simulink model "HybridIntegrationEemshaven"  (R2022b)
settings: Solver=VariableStepAuto  StartTime=0.0  StopTime=1757.5  RelTol=1e-3
undefined symbols (not defined in the file): reactiveCompensationCapacitance
libraries: ee_lib x8, nesl_utility x4, fl_lib x2, spspowerguiLib x1
settings Model: Creator=anton  LastModifiedBy=andreas
settings SolverCC: AlgebraicLoopSolver=TrustRegion
settings DebuggingCC: UnconnectedInputMsg=warning  UnconnectedOutputMsg=warning  UnconnectedLineMsg=warning  SFMachineParentedDataDiag=warning
settings ModelReferenceCC: EnableRefExpFcnMdlSchedulingChecks=on
settings RTWCC: DLArmComputeVersion=19.05

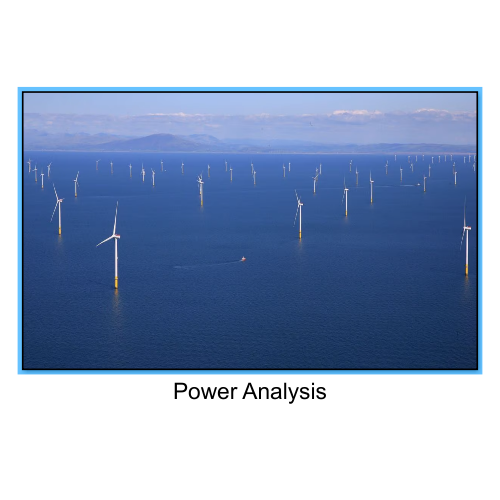
[thumbnail: Simulink's stored preview of the top-level diagram]
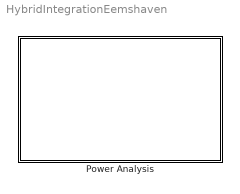
== system HybridIntegrationEemshaven ==
  Power Analysis : Subsystem
      mask Display: image('PowerAnalysis.PNG'); % Use "Edit Image" on toolstrip to change.

== system HybridIntegrationEemshaven/Power Analysis ==
  Ocean Battery : Subsystem
      mask Display: image('OceanBattery.jpg'); % Use "Edit Image" on toolstrip to change.
  Panels Input Data : Subsystem
      mask Display: image('PanelsInputData.jpg'); % Use "Edit Image" on toolstrip to change.
  Production Modules : Subsystem
      mask Display: image('ProductionModules.png'); % Use "Edit Image" on toolstrip to change.
  Scope5 : Scope
  Wave Power Input Data : Subsystem
      mask Display: image('Waves.jpg'); % Use "Edit Image" on toolstrip to change.
  powergui : spspowerguiLib/powergui  Priority=1  SimulationMode=Discrete phasor  SampleTime=0.05  frequency=60  Iterations=50  frequencyindice=60  Pbase=100e6  ErrMax=1e-4  UnitsV=kV  UnitsW=MW  buscounter=0  FunctionMessages=off  echomessages=off  EnableUseOfTLC=off  CurrentSourceSwitches=off  DisableSnubberDevices=off  DisableRonSwitches=off  DisableVfSwitches=off  DisplayEquations=off  AutomaticDiscreteSolvers=off  SolverType=Tustin/Backward Euler (TBE)  Interpol=off  ExternalGateDelay=off  methode=off  Ts=100  x0status=blocks  SPID=on  SwTol=0  HookPort=off  NonlinearTolerance=1e-4  nMaxIteration=100  ContinueOnMaxIteration=off  RestoreLinks=warning  ResistiveCurrentMeasurement=off  Frange=[0:2:500]  Ylog=off  Xlog=on  ShowGrid=off  save=off  variable=ZData  structure=0  ZoomFFT=off  StartTime=0.0  cycles=1  DisplayStyle=1  fundamental=60  FreqAxis=off  MaxFrequency=1000  frequencyindicesteady=1  RmsSteady=1  display=off
  wires:
  Production Modules/1("Total Power (Wind, Sun, Wave)") -> Ocean Battery/1(Input), Scope5/1

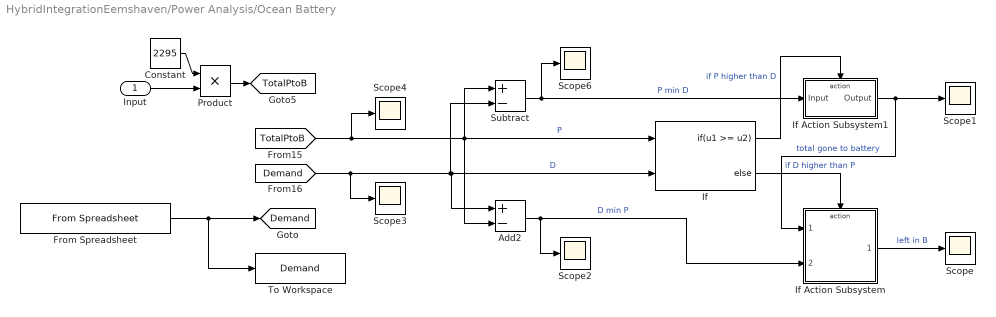
== system HybridIntegrationEemshaven/Power Analysis/Ocean Battery ==
  Input : Inport
  Add2 : Sum  Inputs=+-
  Constant : Constant  Value=2295
  From Spreadsheet : FromSpreadsheet  FileName=Copy of DemandSheet5.xlsx  SheetName=Sheet5  Range=A2:B35654  SampleTime=0.05
  If : If  NumInputs=2  IfExpression=u1 >= u2
  If Action Subsystem : Subsystem  TreatAsAtomicUnit=on
  If Action Subsystem1 : Subsystem  TreatAsAtomicUnit=on
  Product : Product
  Scope{,1..4,6} (6 alike) : Scope
  Subtract : Sum  Inputs=+-
  To Workspace : ToWorkspace  VariableName=Demand  SampleTime=-1
      settings: Save2DSignal=2-D array (concatenate along first dimension)
  tag scope: Demand=global, TotalPtoB=global
  wires:
  [TotalPtoB] -> Scope4/1, Subtract/1, If/1, Add2/2  "P"
  If Action Subsystem/1(Output) -> Scope/1  "left in B"
  Constant/1 -> Product/1
  [Demand] -> Add2/1, If/2, Subtract/2, Scope3/1  "D"
  Add2/1 -> If Action Subsystem/2(D min P), Scope2/1  "D min P"
  Subtract/1 -> If Action Subsystem1/1(Input), Scope6/1  "P min D"
  If Action Subsystem1/1(Output) -> If Action Subsystem/1(Total to battery), Scope1/1  "total gone to battery"
  From Spreadsheet/1 -> To Workspace/1, [Demand]
  If/2 -> If Action Subsystem/Action  "if D higher than P"
  Product/1 -> [TotalPtoB]
  Input/1 -> Product/2
  If/1 -> If Action Subsystem1/Action  "if P higher than D"

== system HybridIntegrationEemshaven/Power Analysis/Panels Input Data ==
  From Spreadsheet : FromSpreadsheet  FileName=EemshavenVoltageSheet4.xlsx  SheetName=Sheet4  Range=A2:B35300  SampleTime=0.05
  From Spreadsheet1 : FromSpreadsheet  FileName=EemshavenSunIrradSheet5.xlsx  SheetName=Sheet5  Range=A2:B35300  SampleTime=0.05
  Scope1 : Scope
  Scope2 : Scope
  tag scope: G=global, Voltage=global
  wires:
  From Spreadsheet1/1 -> Scope1/1, [G]
  From Spreadsheet/1 -> [Voltage], Scope2/1

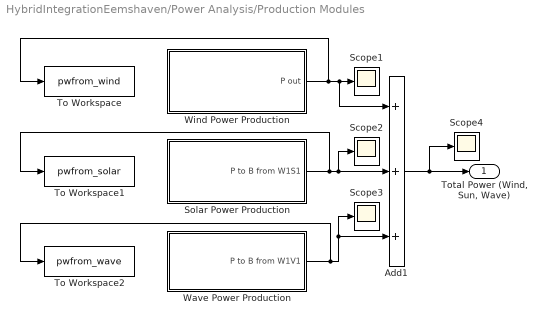
== system HybridIntegrationEemshaven/Power Analysis/Production Modules ==
  Add1 : Sum  Inputs=+++
  Scope{1..4} (4 alike) : Scope
  Solar Power Production : Subsystem
      mask Display: image('Panels.jpg'); % Use "Edit Image" on toolstrip to change.
  To Workspace : ToWorkspace  VariableName=pwfrom_wind  SampleTime=0.05
      settings: Save2DSignal=2-D array (concatenate along first dimension)
  To Workspace1 : ToWorkspace  VariableName=pwfrom_solar  SampleTime=-1
      settings: Save2DSignal=2-D array (concatenate along first dimension)
  To Workspace2 : ToWorkspace  VariableName=pwfrom_wave  SampleTime=-1
      settings: Save2DSignal=2-D array (concatenate along first dimension)
  Wave Power Production : Subsystem
      mask Display: image('WavePower.jpeg'); % Use "Edit Image" on toolstrip to change.
  Wind Power Production : Subsystem
      mask Display: image('WindPower.PNG'); % Use "Edit Image" on toolstrip to change.
  "Total Power (Wind, Sun, Wave)" : Outport
  wires:
  Add1/1 -> "Total Power (Wind, Sun, Wave)"/1, Scope4/1
  Solar Power Production/1(P to B from W1S1) -> To Workspace1/1, Add1/2, Scope2/1
  Wind Power Production/1(P out) -> Add1/1, Scope1/1, To Workspace/1
  Wave Power Production/1(P to B from W1V1) -> To Workspace2/1, Scope3/1, Add1/3

== system HybridIntegrationEemshaven/Power Analysis/Wave Power Input Data ==
  From Spreadsheet : FromSpreadsheet  FileName=EemshavenWavePerBuoySheet5.xlsx  SheetName=Sheet5  Range=A2:B35533  SampleTime=0.05
  tag scope: WavePower=global
  wires:
  From Spreadsheet/1 -> [WavePower]

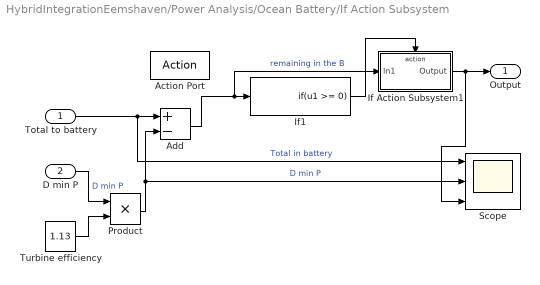
== system HybridIntegrationEemshaven/Power Analysis/Ocean Battery/If Action Subsystem ==
  Total to battery : Inport
  D min P : Inport  Port=2
  Action Port : ActionPort  ActionPortLabel=else
  Add : Sum  Inputs=+-
  If Action Subsystem1 : Subsystem  TreatAsAtomicUnit=on
  If1 : If  IfExpression=u1 >= 0  ShowElse=off
  Product : Product
  Scope : Scope  NumInputPorts=3
  Turbine efficiency : Constant  Value=1.13
  Output : Outport
  wires:
  D min P/1 -> Product/1  "D min P"
  Product/1 -> Add/2, Scope/2  "D min P"
  Total to battery/1 -> Add/1, Scope/1  "Total in battery"
  Turbine efficiency/1 -> Product/2
  If1/1 -> If Action Subsystem1/Action
  Add/1 -> If Action Subsystem1/1(In1), If1/1  "remaining in the B"
  If Action Subsystem1/1(Output) -> Scope/3, Output/1

== system HybridIntegrationEemshaven/Power Analysis/Ocean Battery/If Action Subsystem1 ==
  Input : Inport
  Action Port : ActionPort  ActionPortLabel=if(u1 >= u2)
  If Action Subsystem1 : Subsystem  TreatAsAtomicUnit=on
  If1 : If  IfExpression=u1 <= 2.44e+6  ShowElse=off
  Scope : Scope
  Output : Outport
  wires:
  Input/1 -> If Action Subsystem1/1(Input), If1/1  "To Battery"
  If Action Subsystem1/1(Output) -> Scope/1, Output/1
  If1/1 -> If Action Subsystem1/Action

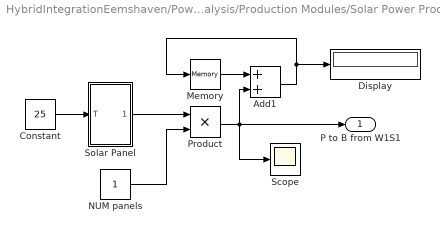
== system HybridIntegrationEemshaven/Power Analysis/Production Modules/Solar Power Production ==
  Add1 : Sum
  Constant : Constant  Value=25
  Display : Display
  Memory : Memory
  NUM panels : Constant
  Product : Product
  Scope : Scope
  Solar Panel : Subsystem
  P to B from W1S1 : Outport
  wires:
  Constant/1 -> Solar Panel/1(T)
  Product/1 -> Scope/1, Add1/2, P to B from W1S1/1
  NUM panels/1 -> Product/2
  Solar Panel/1(Out1) -> Product/1
  Add1/1 -> Memory/1, Display/1
  Memory/1 -> Add1/1

== system HybridIntegrationEemshaven/Power Analysis/Production Modules/Wave Power Production ==
  NUM_buoys : Constant
  Product : Product
  Scope16 : Scope
  P to B from W1V1 : Outport
  wires:
  NUM_buoys/1 -> Product/1
  [WavePower] -> Product/2
  Product/1 -> Scope16/1, P to B from W1V1/1

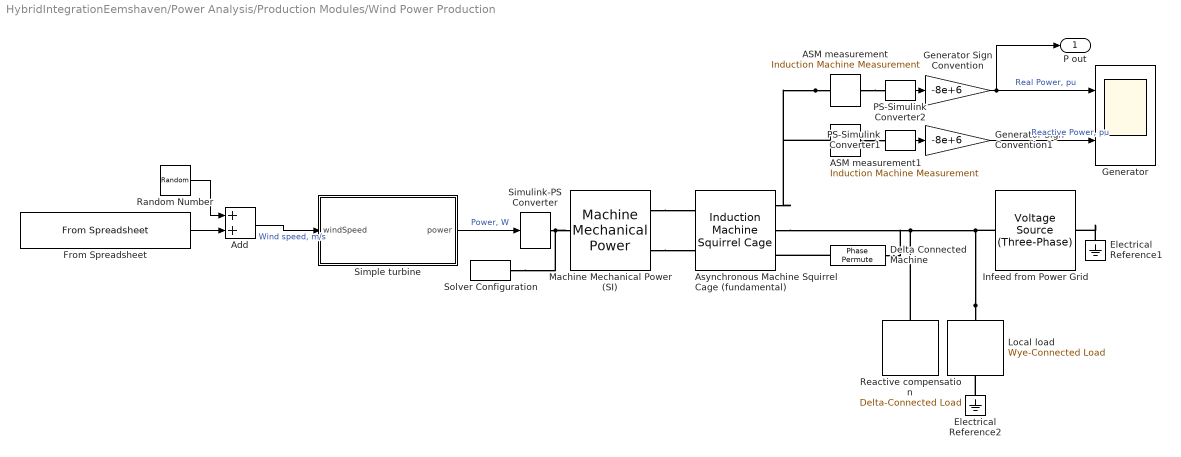
== system HybridIntegrationEemshaven/Power Analysis/Production Modules/Wind Power Production ==
  ASM measurement : ee_lib/Electromechanical/Asynchronous/Induction Machine Measurement  output_idx=11
      settings: InternalSimscapePortConfiguration="{\"Bottom\":[],\"Left\":[{\"id\":\"pu_input\",\"label\":\"pu\",\"type\":\"input\"}],\"Right\":[{\"id\":\"pu_output\",\"label\":\"o\",\"type\":\"output\"}],\"Top\":[]}"
  ASM measurement1 : ee_lib/Electromechanical/Asynchronous/Induction Machine Measurement  output_idx=12
      settings: InternalSimscapePortConfiguration="{\"Bottom\":[],\"Left\":[{\"id\":\"pu_input\",\"label\":\"pu\",\"type\":\"input\"}],\"Right\":[{\"id\":\"pu_output\",\"label\":\"o\",\"type\":\"output\"}],\"Top\":[]}"
  Add : Sum
  Asynchronous Machine Squirrel Cage (fundamental) : ee_lib/Electromechanical/Asynchronous/Induction Machine Squirrel Cage  port_option=ee.enum.threePhasePort.composite  SRated=SRated V*A  VRated=VRated V  FRated=FRated Hz  nPolePairs=2  param_unit=ee.enum.unit.si  squirrel_cage=ee.enum.squirrelcage.Single  zero_sequence=ee.enum.park.zerosequence.include  initialization_option=ee.enum.asm.initialization.fluxvariables  Rs=0.25 Ohm  Xls=0.4 Ohm  pu_Rs=0.0258  pu_Lls=0.0413  Rrd=0.14 Ohm  Xlrd=0.41 Ohm  pu_Rrd=0.0145  pu_Llrd=0.0424  Rrd1=0.28 Ohm  Xlrd1=0.82 Ohm  Rrd2=0.28 Ohm  Xlrd2=0.82 Ohm  pu_Rrd1=0.0290  pu_Llrd1=0.0848  pu_Rrd2=0.0290  pu_Llrd2=0.0848  Xm=17 Ohm  pu_Lm=1.7562  X0=0.4 Ohm  pu_L0=0.0413  saturation_option=ee.enum.saturation.exclude  saturation_i=[0, 4, 9, 18, 25, 34, 50, 68, 95, 120] A  saturation_v=[0, 88, 154, 198, 220, 242, 264, 286, 308, 327] V  pu_saturation_i=[0, .176, .396, .792, 1.1, 1.496, 2.2, 2.992, 4.18, 5.28]  pu_saturation_v=[0, .4, .7, .9, 1, 1.1, 1.2, 1.3, 1.4, 1.4864]  connection_option=ee.enum.Connection.delta1  angular_position_specify=off  angular_position_priority=None  angular_position=0 deg  angular_position_nominal_specify=off  angular_position_nominal_unit=deg  angular_position_nominal_value=1  pu_psids_specify=off  pu_psids_priority=None  pu_psids=0  pu_psids_nominal_specify=off  pu_psids_nominal_unit=1  pu_psids_nominal_value=1  pu_psiqs_specify=off  pu_psiqs_priority=None  pu_psiqs=0  pu_psiqs_nominal_specify=off  pu_psiqs_nominal_unit=1  pu_psiqs_nominal_value=1  pu_psi0s_specify=off  pu_psi0s_priority=None  pu_psi0s=0  pu_psi0s_nominal_specify=off  pu_psi0s_nominal_unit=1  pu_psi0s_nominal_value=1  pu_psidr_specify=off  pu_psidr_priority=None  pu_psidr=0  pu_psidr_nominal_specify=off  pu_psidr_nominal_unit=1  pu_psidr_nominal_value=1  pu_psiqr_specify=off  pu_psiqr_priority=None  pu_psiqr=0  pu_psiqr_nominal_specify=off  pu_psiqr_nominal_unit=1  pu_psiqr_nominal_value=1  pu_psidr1_specify=off  pu_psidr1_priority=None  pu_psidr1=0  pu_psidr1_nominal_specify=off  pu_psidr1_nominal_unit=1  pu_psidr1_nominal_value=1  pu_psiqr1_specify=off  pu_psiqr1_priority=None  pu_psiqr1=0  pu_psiqr1_nominal_specify=off  pu_psiqr1_nominal_unit=1  pu_psiqr1_nominal_value=1  pu_psidr2_specify=off  pu_psidr2_priority=None  pu_psidr2=0  pu_psidr2_nominal_specify=off  pu_psidr2_nominal_unit=1  pu_psidr2_nominal_value=1  pu_psiqr2_specify=off  pu_psiqr2_priority=None  pu_psiqr2=0  pu_psiqr2_nominal_specify=off  pu_psiqr2_nominal_unit=1  pu_psiqr2_nominal_value=1  psids_specify=off  psids_priority=None  psids=0 Wb  psids_nominal_specify=off  psids_nominal_unit=Wb  psids_nominal_value=1  psiqs_specify=off  psiqs_priority=None  psiqs=0 Wb  psiqs_nominal_specify=off  psiqs_nominal_unit=Wb  psiqs_nominal_value=1  psi0s_specify=off  psi0s_priority=None  psi0s=0 Wb  psi0s_nominal_specify=off  psi0s_nominal_unit=Wb  psi0s_nominal_value=1  psidr_specify=off  psidr_priority=None  psidr=0 Wb  psidr_nominal_specify=off  psidr_nominal_unit=Wb  psidr_nominal_value=1  psiqr_specify=off  psiqr_priority=None  psiqr=0 Wb  psiqr_nominal_specify=off  psiqr_nominal_unit=Wb  psiqr_nominal_value=1  psidr1_specify=off  psidr1_priority=None  psidr1=0 Wb  psidr1_nominal_specify=off  psidr1_nominal_unit=Wb  psidr1_nominal_value=1  psiqr1_specify=off  psiqr1_priority=None  psiqr1=0 Wb  psiqr1_nominal_specify=off  psiqr1_nominal_unit=Wb  psiqr1_nominal_value=1  psidr2_specify=off  psidr2_priority=None  psidr2=0 Wb  psidr2_nominal_specify=off  psidr2_nominal_unit=Wb  psidr2_nominal_value=1  psiqr2_specify=off  psiqr2_priority=None  psiqr2=0 Wb  psiqr2_nominal_specify=off  psiqr2_nominal_unit=Wb  psiqr2_nominal_value=1  slip_specify=off  slip_priority=None  slip=0  slip_nominal_specify=off  slip_nominal_unit=1  slip_nominal_value=1  real_power_generated_specify=off  real_power_generated_priority=None  real_power_generated=0 W  real_power_generated_nominal_specify=off  real_power_generated_nominal_unit=W  real_power_generated_nominal_value=1  mechanical_power_consumed_specify=off  mechanical_power_consumed_priority=None  mechanical_power_consumed=0 W  mechanical_power_consumed_nominal_specify=off  mechanical_power_consumed_nominal_unit=W  mechanical_power_consumed_nominal_value=1  Tmeas=298.15 K  alpha=3.93e-3 1/K  alpha_cage=4.4e-3 1/K  stator_thermal_mass=100 J/K  rotor_thermal_mass=200 J/K  temperatureA_specify=off  temperatureA_priority=High  temperatureA=25 degC  temperatureA_nominal_specify=off  temperatureA_nominal_unit=degC  temperatureA_nominal_value=1  temperatureB_specify=off  temperatureB_priority=High  temperatureB=25 degC  temperatureB_nominal_specify=off  temperatureB_nominal_unit=degC  temperatureB_nominal_value=1  temperatureC_specify=off  temperatureC_priority=High  temperatureC=25 degC  temperatureC_nominal_specify=off  temperatureC_nominal_unit=degC  temperatureC_nominal_value=1  temperatureR_specify=off  temperatureR_priority=High  temperatureR=25 degC  temperatureR_nominal_specify=off  temperatureR_nominal_unit=degC  temperatureR_nominal_value=1
      settings: InternalSimscapePortConfiguration="{\"Bottom\":[],\"Left\":[{\"id\":\"R\",\"label\":\"R\",\"type\":\"foundation.mechanical.rotational.rotational\"},{\"id\":\"C\",\"label\":\"C\",\"type\":\"foundation.mechanical.rotational.rotational\"}],\"Right\":[{\"id\":\"pu_output\",\"label\":\"pu\",\"type\":\"output\"},{\"id\":\"N1\",\"label\":\"~1\",\"type\":\"foundation.electrical.three_phase\"},{\"id\":\"N2\",\"label\":\"~2\",\"type\":\"foundation.electrical.three_phase\"}],\"Top\":[]}"
  Delta Connected Machine : ee_lib/Connectors & References/Phase Permute
      settings: InternalSimscapePortConfiguration="{\"Bottom\":[],\"Left\":[{\"id\":\"N123\",\"label\":\"~123\",\"type\":\"foundation.electrical.three_phase\"}],\"Right\":[{\"id\":\"N231\",\"label\":\"~231\",\"type\":\"foundation.electrical.three_phase\"}],\"Top\":[]}"
  Electrical Reference1 : fl_lib/Electrical/Electrical Elements/Electrical Reference
  Electrical Reference2 : fl_lib/Electrical/Electrical Elements/Electrical Reference
  From Spreadsheet : FromSpreadsheet  FileName=EemshavenWindspeedSheet6.xlsx  SheetName=Sheet6  Range=A2:B35170  SampleTime=0.05
  Generator : Scope  NumInputPorts=2
  Generator Sign Convention : Gain  Gain=-8e+6
  Generator Sign Convention1 : Gain  Gain=-8e+6
  Infeed from Power Grid : ee_lib/Sources/Voltage Source (Three-Phase)  vline_rms=VRated V  shift=0 deg  freq=FRated Hz  impedance_option=0  SShortCircuit=1e6 V*A  XR=15  R=0.01 Ohm  L=3.97e-4 H  harmonic_option=0  harmonic_orders=[5, 7, 11, 13]  harmonic_ratios=[0.1, 0.1, 0.1, 0.1]  G_parasitic=0 1/Ohm  I_specify=off  I_priority=None  I=[ 0 0 0 ] A  I_nominal_specify=off  I_nominal_unit=A  I_nominal_value=1
  Local load : ee_lib/Passive/RLC Assemblies/Wye-Connected Load  parameterization=2  component_structure=1  component_structure_PQ=1  R=1 Ohm  L=0.001 H  C=1e-6 F  VRated=VRated V  FRated=60 Hz  P=75e3 W  Qpos=100 V*A  Qneg=-100 V*A  R_parasitic=1e-6 Ohm  G_parasitic=1e-6 1/Ohm  R_parasitic_PQ=1e-6 Ohm  G_parasitic_PQ=1e-6 1/Ohm  Vmag0=2.4e+4 V  Vang0=0 deg  Freq0=60 Hz  IL_specify=on  IL_priority=High  IL=[ 0 0 0 ] A  IL_nominal_specify=off  IL_nominal_unit=A  IL_nominal_value=1  VC_specify=on  VC_priority=High  VC=[ 0 0 0 ] V  VC_nominal_specify=off  VC_nominal_unit=V  VC_nominal_value=1
  Machine Mechanical Power (SI) : ee_lib/Electromechanical/Mechanical/Machine Mechanical Power  power_sign=-1  SRated=SRated V*A  FRated=FRated Hz  nPolePairs=2  inputUnit=ee.enum.unit.si  torque_factor=2  inertia_option=2  J=27548 kg*m^2  H=4 s*W/V/A  damper_option=2  D=39.0509 N*m/(rad/s)  pu_D=0.01  initialization_option=2  fMechanical0=30 Hz  fElectrical0=FRated Hz
      settings: InternalSimscapePortConfiguration="{\"Bottom\":[],\"Left\":[{\"id\":\"Pm\",\"label\":\"Pm\",\"type\":\"input\"}],\"Right\":[{\"id\":\"R\",\"label\":\"R\",\"type\":\"foundation.mechanical.rotational.rotational\"},{\"id\":\"C\",\"label\":\"C\",\"type\":\"foundation.mechanical.rotational.rotational\"}],\"Top\":[]}"
  PS-Simulink Converter1 : nesl_utility/PS-Simulink Converter  PhysicalDomain=network_engine_domain  SubClassName=ps_output  LeftPortType=input  RightPortType=output  PseudoPeriodic=off  Frequencies=[]  VectorFormat=1-D array  Unit=1  AffineConversion=off
  PS-Simulink Converter2 : nesl_utility/PS-Simulink Converter  PhysicalDomain=network_engine_domain  SubClassName=ps_output  LeftPortType=input  RightPortType=output  PseudoPeriodic=off  Frequencies=[]  VectorFormat=1-D array  Unit=1  AffineConversion=off
  Random Number : RandomNumber  Mean=5  Variance=3  SampleTime=0.05
  Reactive compensation : ee_lib/Passive/RLC Assemblies/Delta-Connected Load  parameterization=1  component_structure=3  component_structure_PQ=1  R=1 Ohm  L=0.001 H  C=reactiveCompensationCapacitance F  VRated=2.4e+4 V  FRated=60 Hz  P=1000 W  Qpos=100 V*A  Qneg=-100 V*A  R_parasitic=1e-6 Ohm  G_parasitic=1e-6 1/Ohm  R_parasitic_PQ=1e-6 Ohm  G_parasitic_PQ=1e-6 1/Ohm  Vmag0=2.4e+4 V  Vang0=0 deg  Freq0=60 Hz  IL_specify=on  IL_priority=High  IL=[ 0 0 0 ] A  IL_nominal_specify=off  IL_nominal_unit=A  IL_nominal_value=1  VC_specify=on  VC_priority=High  VC=[ 0 0 0 ] V  VC_nominal_specify=off  VC_nominal_unit=V  VC_nominal_value=1
      settings: InternalSimscapePortConfiguration="{\"Bottom\":[],\"Left\":[{\"id\":\"N\",\"label\":\"~\",\"type\":\"foundation.electrical.three_phase\"}],\"Right\":[],\"Top\":[]}"
  Simple turbine : MATLAB Function  TreatAsAtomicUnit=on  mask(Simple Turbine){ratedOutputPower=150e3, cutInSpeed=3, ratedOutputSpeed=12, cutOutSpeed=23}
      mask prompts: ratedOutputPower "Rated output power, W"; cutInSpeed "Cut-in speed, m/s"; ratedOutputSpeed "Rated output speed, m/s"; cutOutSpeed "Cut-out speed, m/s"
      mask help:
      | This function implements a simple power versus wind speed characteristic to represent a wind turbine.
      |
      | Given an input of wind speed, m/s, the function outputs turbine power, W.
      |
      | The parameters must meet the following requirement:
      |
      | Cut-in speed < Rated output speed < Cut-out speed
  Simulink-PS Converter : nesl_utility/Simulink-PS Converter  PhysicalDomain=network_engine_domain  SubClassName=ps_input  LeftPortType=input  RightPortType=output  PseudoPeriodic=off  Frequencies=[]  NoiseDistribution=none  NoiseParameters=[]  Unit=1  AffineConversion=off  FilteringAndDerivatives=zero  SimscapeFilterOrder=1  InputFilterTimeConstant=0.001  UdotUserProvided=1
  Solver Configuration : nesl_utility/Solver Configuration  PhysicalDomain=network_engine_domain  SubClassName=solver  LeftPortType=input  RightPortType=generic  Tones=[]  Harmonics=[]  SimulateNoise=off  Profile=off  UseLocalSampling=off  EnableSwitchedLinearOptims=on  FrequencyDomain=off  UseCCode=off  RelTol=0.001  AbsTol=1e-06  MinStep=1e-09  ToWorkspace=off  RevertToSquareIcSolve=off  NumHomotopyIterations=100  PhasorMode=off  PhasorModeNumHarmonics=1  ConsistencySolver=NEWTON_FTOL  IndexReductionMethod=DerivativeReplacement  DoDC=off  ResidualTolerance=1e-9  ConsistencyTolSource=GLOBAL  ConsistencyAbsTol=0.001  ConsistencyRelTol=0.001  ConsistencyTolFactor=0.001  UseLocalSolver=on  LocalSolverChoice=NE_BACKWARD_EULER_ADVANCER  ResolveIndetEquations=on  FunctionEvalNumThread=1  LocalSolverSampleTime=1e-3  DoFixedCost=on  MaxNonlinIter=3  MaxModeIter=2  ComputeImpulses=off  ImpulseIterations=2  LinearAlgebra=auto  LinearAlgebraNumThread=0  EquationFormulation=NE_TIME_EF  DelaysMemoryBudget=1024  AutomaticFiltering=on  FilteringTimeConstant=0.001  PartitionStorageMethod=AS_NEEDED  PartitionMemoryBudget=1024  PartitionMethod=FAST
  P out : Outport
  wires:
  ? -> ?
  Generator Sign Convention1/1 -> Generator/2  "Reactive Power, pu"
  Simple turbine/1(power) -> Simulink-PS Converter/1  "Power, W"
  Generator Sign Convention/1 -> P out/1, Generator/1  "Real Power, pu"
  PS-Simulink Converter1/1 -> Generator Sign Convention1/1
  PS-Simulink Converter2/1 -> Generator Sign Convention/1
  From Spreadsheet/1 -> Add/2
  Random Number/1 -> Add/1
  Add/1 -> Simple turbine/1(windSpeed)  "Wind speed, m/s"
  connections:
  Simulink-PS Converter/RConn1 -- Machine Mechanical Power (SI)/LConn1 -- Solver Configuration/RConn1
  ASM measurement/LConn1 -- Asynchronous Machine Squirrel Cage (fundamental)/RConn1 -- ASM measurement1/LConn1
  Local load/LConn1 -- Infeed from Power Grid/RConn1 -- Asynchronous Machine Squirrel Cage (fundamental)/RConn2 -- Delta Connected Machine/LConn1 -- Reactive compensation/LConn1
  Machine Mechanical Power (SI)/RConn1 -- Asynchronous Machine Squirrel Cage (fundamental)/LConn1
  ASM measurement/RConn1 -- PS-Simulink Converter2/LConn1
  Electrical Reference1/LConn1 -- Infeed from Power Grid/LConn1
  Delta Connected Machine/RConn1 -- Asynchronous Machine Squirrel Cage (fundamental)/RConn3
  ASM measurement1/RConn1 -- PS-Simulink Converter1/LConn1
  Electrical Reference2/LConn1 -- Local load/RConn1
  Machine Mechanical Power (SI)/RConn2 -- Asynchronous Machine Squirrel Cage (fundamental)/LConn2

== system HybridIntegrationEemshaven/Power Analysis/Ocean Battery/If Action Subsystem/If Action Subsystem1 ==
  In1 : Inport
  Action Port : ActionPort  ActionPortLabel=if(u1 >= 0)
  Output : Outport
  wires:
  In1/1 -> Output/1

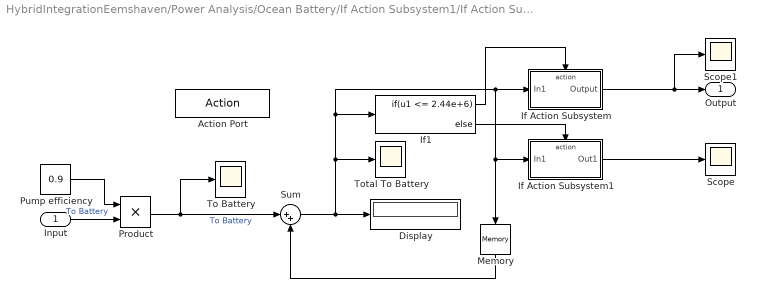
== system HybridIntegrationEemshaven/Power Analysis/Ocean Battery/If Action Subsystem1/If Action Subsystem1 ==
  Input : Inport
  Action Port : ActionPort  ActionPortLabel=if(u1 <= 2.44e+6)
  Display : Display
  If Action Subsystem : Subsystem  TreatAsAtomicUnit=on
  If Action Subsystem1 : Subsystem  TreatAsAtomicUnit=on
  If1 : If  IfExpression=u1 <= 2.44e+6
  Memory : Memory  InheritSampleTime=on
  Product : Product
  Pump efficiency : Constant  Value=0.9
  Scope : Scope
  Scope1 : Scope
  Sum : Sum  Inputs=|++
  To Battery : Scope
  Total To Battery : Scope
  Output : Outport
  wires:
  Pump efficiency/1 -> Product/1
  Input/1 -> Product/2  "To Battery"
  Product/1 -> Sum/1, To Battery/1  "To Battery"
  Memory/1 -> Sum/2
  If Action Subsystem/1(Output) -> Output/1, Scope1/1
  If Action Subsystem1/1(Out1) -> Scope/1
  If1/2 -> If Action Subsystem1/Action
  Sum/1 -> Display/1, If Action Subsystem/1(In1), If Action Subsystem1/1(In1), Memory/1, If1/1, Total To Battery/1
  If1/1 -> If Action Subsystem/Action

== system HybridIntegrationEemshaven/Power Analysis/Production Modules/Solar Power Production/Solar Panel ==
  T : Inport
  PV Module : Subsystem
  Product : Product
  Scope : Scope
  Voltage : Scope
  Out1 : Outport
  wires:
  T/1 -> PV Module/1(T)
  PV Module/2(I) -> Product/2
  PV Module/1(V) -> Product/1, Voltage/1
  Product/1 -> Scope/1, Out1/1

== system HybridIntegrationEemshaven/Power Analysis/Ocean Battery/If Action Subsystem1/If Action Subsystem1/If Action Subsystem ==
  In1 : Inport
  Action Port : ActionPort  ActionPortLabel=if(u1 <= 2.44e+6)
  Output : Outport
  wires:
  In1/1 -> Output/1

== system HybridIntegrationEemshaven/Power Analysis/Ocean Battery/If Action Subsystem1/If Action Subsystem1/If Action Subsystem1 ==
  In1 : Inport
  Action Port : ActionPort  ActionPortLabel=else
  Out1 : Outport
  wires:
  In1/1 -> Out1/1

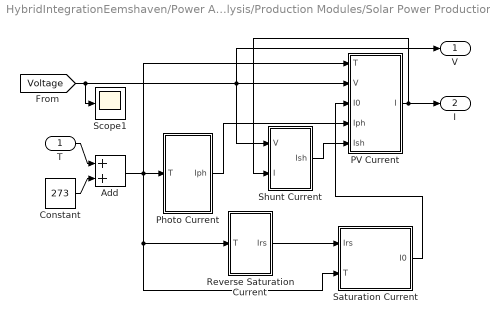
== system HybridIntegrationEemshaven/Power Analysis/Production Modules/Solar Power Production/Solar Panel/PV Module ==
  T : Inport
  Add : Sum
  Constant : Constant  Value=273
  PV Current : Subsystem
  Photo Current : Subsystem
  Reverse Saturation Current : Subsystem
  Saturation Current : Subsystem
  Scope1 : Scope
  Shunt Current : Subsystem
  V : Outport
  I : Outport  Port=2
  wires:
  Saturation Current/1(I0) -> PV Current/3(I0)
  Add/1 -> PV Current/1(T), Saturation Current/2(T), Reverse Saturation Current/1(T), Photo Current/1(T)
  T/1 -> Add/1
  Reverse Saturation Current/1(Irs) -> Saturation Current/1(Irs)
  Photo Current/1(Iph) -> PV Current/4(Iph)
  PV Current/1(I) -> I/1, Shunt Current/2(I)
  [Voltage] -> Scope1/1, Shunt Current/1(V), PV Current/2(V), V/1
  Shunt Current/1(Ish) -> PV Current/5(Ish)
  Constant/1 -> Add/2

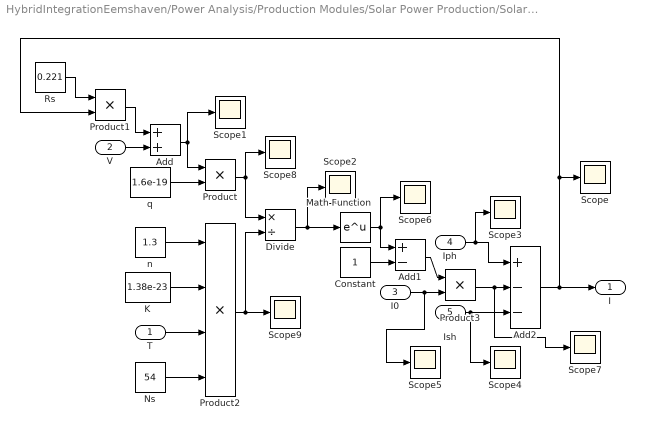
== system HybridIntegrationEemshaven/Power Analysis/Production Modules/Solar Power Production/Solar Panel/PV Module/PV Current ==
  T : Inport
  V : Inport  Port=2
  I0 : Inport  Port=3
  Iph : Inport  Port=4
  Ish : Inport  Port=5
  Add : Sum
  Add1 : Sum  Inputs=+-
  Add2 : Sum  Inputs=+--
  Constant : Constant
  Divide : Product  Inputs=*/
  K : Constant  Value=1.38e-23
  Math Function : Math
  Ns : Constant  Value=54
  Product : Product
  Product1 : Product
  Product2 : Product  Inputs=4
  Product3 : Product
  Rs : Constant  Value=0.221
  Scope{,1..9} (10 alike) : Scope
  n : Constant  Value=1.3
  q : Constant  Value=1.6e-19
  I : Outport
  wires:
  I0/1 -> Scope5/1, Product3/2
  Add2/1 -> Scope/1, Product1/2, I/1
  n/1 -> Product2/1
  Constant/1 -> Add1/2
  Add/1 -> Product/1, Scope1/1
  Divide/1 -> Scope2/1, Math Function/1
  Add1/1 -> Product3/1
  Rs/1 -> Product1/1
  Product3/1 -> Scope7/1, Add2/2
  V/1 -> Add/2
  T/1 -> Product2/3
  Iph/1 -> Scope3/1, Add2/1
  q/1 -> Product/2
  K/1 -> Product2/2
  Product1/1 -> Add/1
  Math Function/1 -> Scope6/1, Add1/1
  Ns/1 -> Product2/4
  Ish/1 -> Scope4/1, Add2/3
  Product/1 -> Divide/1, Scope8/1
  Product2/1 -> Scope9/1, Divide/2

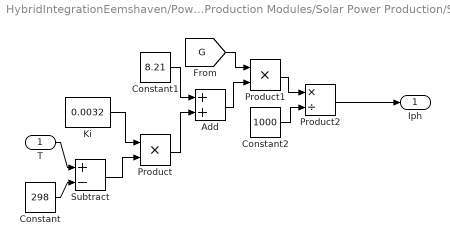
== system HybridIntegrationEemshaven/Power Analysis/Production Modules/Solar Power Production/Solar Panel/PV Module/Photo Current ==
  T : Inport
  Add : Sum
  Constant : Constant  Value=298
  Constant1 : Constant  Value=8.21
  Constant2 : Constant  Value=1000
  Ki : Constant  Value=0.0032
  Product : Product
  Product1 : Product
  Product2 : Product  Inputs=*/
  Subtract : Sum  Inputs=+-
  Iph : Outport
  wires:
  Product2/1 -> Iph/1
  Constant2/1 -> Product2/2
  Subtract/1 -> Product/2
  Constant1/1 -> Add/1
  Ki/1 -> Product/1
  T/1 -> Subtract/1
  Product/1 -> Add/2
  Constant/1 -> Subtract/2
  Add/1 -> Product1/2
  Product1/1 -> Product2/1
  [G] -> Product1/1

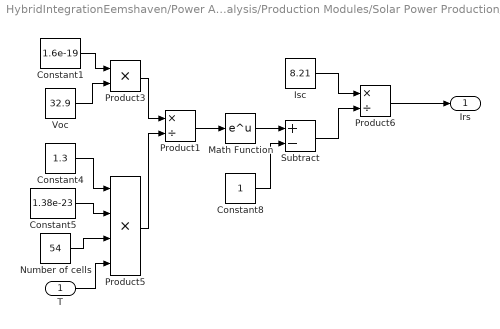
== system HybridIntegrationEemshaven/Power Analysis/Production Modules/Solar Power Production/Solar Panel/PV Module/Reverse Saturation Current ==
  T : Inport
  Constant1 : Constant  Value=1.6e-19
  Constant4 : Constant  Value=1.3
  Constant5 : Constant  Value=1.38e-23
  Constant8 : Constant
  Isc : Constant  Value=8.21
  Math Function : Math
  Number of cells : Constant  Value=54
  Product1 : Product  Inputs=*/
  Product3 : Product
  Product5 : Product  Inputs=4
  Product6 : Product  Inputs=*/
  Subtract : Sum  Inputs=+-
  Voc : Constant  Value=32.9
  Irs : Outport
  wires:
  T/1 -> Product5/4
  Product3/1 -> Product1/1
  Number of cells/1 -> Product5/3
  Product5/1 -> Product1/2
  Math Function/1 -> Subtract/1
  Constant8/1 -> Subtract/2
  Constant1/1 -> Product3/1
  Product6/1 -> Irs/1
  Subtract/1 -> Product6/2
  Constant5/1 -> Product5/2
  Isc/1 -> Product6/1
  Constant4/1 -> Product5/1
  Product1/1 -> Math Function/1
  Voc/1 -> Product3/2

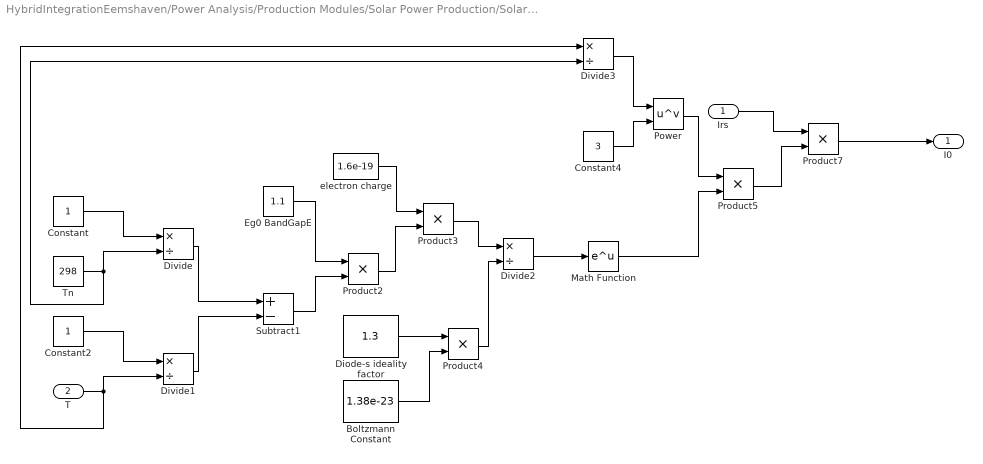
== system HybridIntegrationEemshaven/Power Analysis/Production Modules/Solar Power Production/Solar Panel/PV Module/Saturation Current ==
  Irs : Inport
  T : Inport  Port=2
  Boltzmann Constant : Constant  Value=1.38e-23
  Constant : Constant
  Constant2 : Constant
  Constant4 : Constant  Value=3
  Diode-s ideality factor : Constant  Value=1.3
  Divide{,1..3} (4 alike) : Product  Inputs=*/
  Eg0 BandGapE : Constant  Value=1.1
  Math Function : Math
  Power : Math  Operator=pow
  Product{2..5,7} (5 alike) : Product
  Subtract1 : Sum  Inputs=+-
  Tn : Constant  Value=298
  electron charge : Constant  Value=1.6e-19
  I0 : Outport
  wires:
  Product7/1 -> I0/1
  Product2/1 -> Product3/2
  Divide1/1 -> Subtract1/2
  Constant4/1 -> Power/2
  Divide3/1 -> Power/1
  Constant/1 -> Divide/1
  T/1 -> Divide3/1, Divide1/2
  Irs/1 -> Product7/1
  electron charge/1 -> Product3/1
  Product4/1 -> Divide2/2
  Divide2/1 -> Math Function/1
  Product3/1 -> Divide2/1
  Diode-s ideality factor/1 -> Product4/1
  Subtract1/1 -> Product2/2
  Boltzmann Constant/1 -> Product4/2
  Product5/1 -> Product7/2
  Math Function/1 -> Product5/2
  Eg0 BandGapE/1 -> Product2/1
  Divide/1 -> Subtract1/1
  Tn/1 -> Divide3/2, Divide/2
  Constant2/1 -> Divide1/1
  Power/1 -> Product5/1

== system HybridIntegrationEemshaven/Power Analysis/Production Modules/Solar Power Production/Solar Panel/PV Module/Shunt Current ==
  V : Inport
  I : Inport  Port=2
  Add : Sum
  Product : Product  Inputs=*/
  Product1 : Product
  Series Resistance : Constant  Value=0.221
  Shunt Resistance : Constant  Value=415.405
  Ish : Outport
  wires:
  I/1 -> Product1/2
  Product1/1 -> Add/2
  Shunt Resistance/1 -> Product/2
  Series Resistance/1 -> Product1/1
  V/1 -> Add/1
  Product/1 -> Ish/1
  Add/1 -> Product/1

== matlab function HybridIntegrationEemshaven/Power Analysis/Production Modules/Wind Power Production/Simple turbine ==
  data: windSpeed input; power output; ratedOutputPower parameter; cutInSpeed parameter; ratedOutputSpeed parameter; cutOutSpeed parameter
function power = simpleTurbine( windSpeed, ratedOutputPower, cutInSpeed, ratedOutputSpeed, cutOutSpeed ) %#codegen
%Simple Turbine
% This function implements a simple power versus wind speed characteristic
% to represent a wind turbine.
%
% Given an input of wind speed, m/s, the function outputs turbine power, W.
%
% The parameters must meet the following requirement:
%
% Cut-in speed < Rated output speed < Cut-out speed

% Check rated output power is greater than zero
if ~(ratedOutputPower > 0)
    error( 'Rated output power must be greater than zero.' );
end

% Check cut-in speed is less than rated output speed
if ~(cutInSpeed < ratedOutputSpeed)
    error( 'Cut-in speed must be less than rated output speed.' );
end

% Check rated output speed is less than cut-out speed
if ~(ratedOutputSpeed < cutOutSpeed)
    error( 'Rated output speed must be less than cut-out speed.' );
end

if windSpeed < cutInSpeed
    % Wind speed is less then cut-in speed, power output is zero
    power = 0;
elseif windSpeed < ratedOutputSpeed
    % Wind speed is greater than cut-in speed and less than rated output
    % speed, power output follows linear characteristic from zero to rated
    % power
    cutInGradient = ( ratedOutputPower / ( ratedOutputSpeed - cutInSpeed ) );
    power = cutInGradient * ( windSpeed - cutInSpeed );
elseif windSpeed < cutOutSpeed
    % Wind speed is greater than rated output speed and less than cut-out
    % speed, power output is limited to rated power
    power = ratedOutputPower;
else
    % Wind speed is greater than cut-out speed, power output is zero
    power = 0;
end
